simulink model "Simulation2018_with_Datas"  (R2018b)
settings: Solver=VariableStepAuto  StartTime=0.0  StopTime=10  RelTol=1e-3
undefined symbols (not defined in the file): X, Y, Z
libraries: sm_lib x71, nesl_utility x13
(part 2 of 2)

== matlab function Simulation2018_with_Datas/La acceleration ==
  data: t input; y output
function y = fcn(t)

y=8.262675545e-20*t^13 - 5.538760274e-17*t^12 + 1.650658493e-14*t^11 - 2.882390398e-12*t^10 + 0.0000000003272160959*t^9 - 0.00000002533038828*t^8 + 0.000001364315876*t^7 - 0.00005123490335*t^6 + 0.001324045715*t^5 - 0.02286527605*t^4 + 0.250870264*t^3 - 1.609469938*t^2 + 5.221145819*t - 6.020892607;

== matlab function Simulation2018_with_Datas/LK acceleration ==
  data: t input; y output
function y = fcn(t)

y=4.112469063e-20*t^13 - 2.635696327e-17*t^12 + 7.482039088e-15*t^11 - 1.23869555e-12*t^10 + 0.0000000001325570821*t^9 - 0.000000009607099322*t^8 + 0.0000004806711606*t^7 - 0.00001662975767*t^6 + 0.0003930168135*t^5 - 0.006185334021*t^4 + 0.06218647101*t^3 - 0.371784293*t^2 + 1.124623167*t - 1.153878804;

== matlab function Simulation2018_with_Datas/Ra acceleration ==
  data: t input; y output
function y = fcn(t)

y = 2.639887247e-20*t^13 - 1.911383678e-17*t^12 + 6.106985376e-15*t^11 - 1.135586479e-12*t^10 + 0.0000000001364370212*t^9 - 0.00000001111775708*t^8 + 0.0000006276181862*t^7 - 0.00002464417906*t^6 + 0.0006666026361*t^5 - 0.01213202904*t^4 + 0.1425140779*t^3 - 1.005111791*t^2 + 3.690591562*t - 4.854853304;
